simulink model "Ans_SimulinkEquationModel"  (R2022b)
settings: Solver=VariableStepAuto  StartTime=0.0  StopTime=0.1  RelTol=1e-3
undefined symbols (not defined in the file): C1, L1
settings Model: Creator=ykamatan  LastModifiedBy=ykamatan

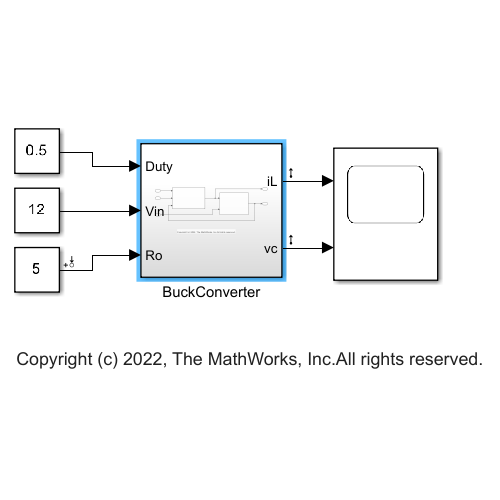
[thumbnail: Simulink's stored preview of the top-level diagram]
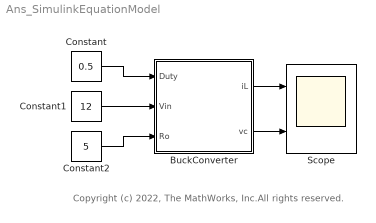
== system Ans_SimulinkEquationModel ==
  note: Copyright (c) 2022, The MathWorks, Inc.All rights reserved.
  BuckConverter : Subsystem
  Constant : Constant  Value=0.5
  Constant1 : Constant  Value=12
  Constant2 : Constant  Value=5
  Scope : Scope  NumInputPorts=2
  wires:
  Constant/1 -> BuckConverter/1(Duty)
  Constant1/1 -> BuckConverter/2(Vin)
  Constant2/1 -> BuckConverter/3(Ro)
  BuckConverter/1(iL) -> Scope/1
  BuckConverter/2(vc) -> Scope/2

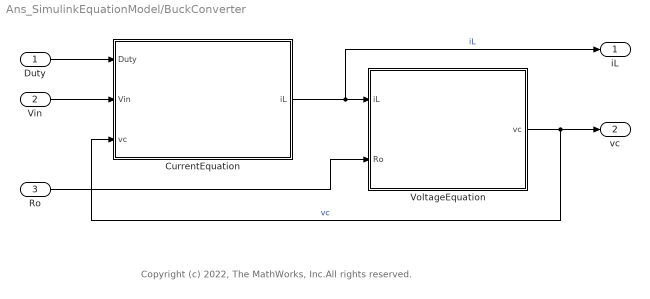
== system Ans_SimulinkEquationModel/BuckConverter ==
  note: Copyright (c) 2022, The MathWorks, Inc.All rights reserved.
  Duty : Inport
  Vin : Inport  Port=2
  Ro : Inport  Port=3
  CurrentEquation : Subsystem
  VoltageEquation : Subsystem
  iL : Outport
  vc : Outport  Port=2
  wires:
  CurrentEquation/1(iL) -> iL/1, VoltageEquation/1(iL)  "iL"
  VoltageEquation/1(vc) -> vc/1, CurrentEquation/3(vc)  "vc"
  Duty/1 -> CurrentEquation/1(Duty)
  Ro/1 -> VoltageEquation/2(Ro)
  Vin/1 -> CurrentEquation/2(Vin)

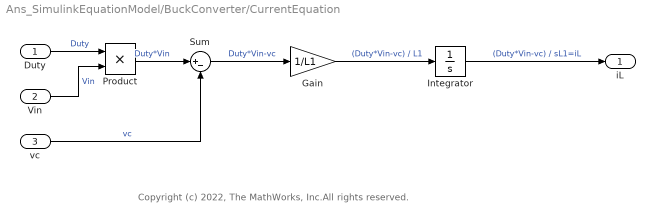
== system Ans_SimulinkEquationModel/BuckConverter/CurrentEquation ==
  note: Copyright (c) 2022, The MathWorks, Inc.All rights reserved.
  Duty : Inport
  Vin : Inport  Port=2
  vc : Inport  Port=3
  Gain : Gain  Gain=1/L1
  Integrator : Integrator
  Product : Product
  Sum : Sum  Inputs=|+-
  iL : Outport
  wires:
  Integrator/1 -> iL/1  "(Duty*Vin-vc) / sL1=iL"
  Gain/1 -> Integrator/1  "(Duty*Vin-vc) / L1"
  Duty/1 -> Product/1  "Duty"
  Vin/1 -> Product/2  "Vin"
  Product/1 -> Sum/1  "Duty*Vin"
  vc/1 -> Sum/2  "vc"
  Sum/1 -> Gain/1  "Duty*Vin-vc"

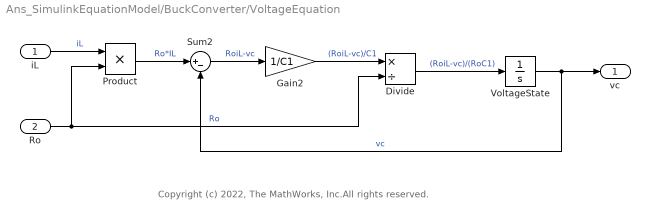
== system Ans_SimulinkEquationModel/BuckConverter/VoltageEquation ==
  note: Copyright (c) 2022, The MathWorks, Inc.All rights reserved.
  iL : Inport
  Ro : Inport  Port=2
  Divide : Product  Inputs=*/
  Gain2 : Gain  Gain=1/C1
  Product : Product
  Sum2 : Sum  Inputs=|+-
  VoltageState : Integrator
  vc : Outport
  wires:
  VoltageState/1 -> Sum2/2, vc/1  "vc"
  Gain2/1 -> Divide/1  "(RoiL-vc)/C1"
  Sum2/1 -> Gain2/1  "RoiL-vc"
  iL/1 -> Product/1  "iL"
  Product/1 -> Sum2/1  "Ro*IL"
  Ro/1 -> Divide/2, Product/2  "Ro"
  Divide/1 -> VoltageState/1  "(RoiL-vc)/(RoC1)"
